simulink model "runQP"  (R2018a)
settings: Solver=VariableStepAuto  StartTime=0.0  StopTime=simTime  RelTol=1e-3
values from neighbouring files (symbols this model uses):
  Kd = 10    [com_notc.m]
  Kp = 200    [com_notc.m]
  q_initial_pos = robot.homeConfiguration    [com_notc.m]
undefined symbols (not defined in the file or in its folder): com_initial_pos
settings Model: Creator=yyakupoglu  LastModifiedBy=yyakupoglu

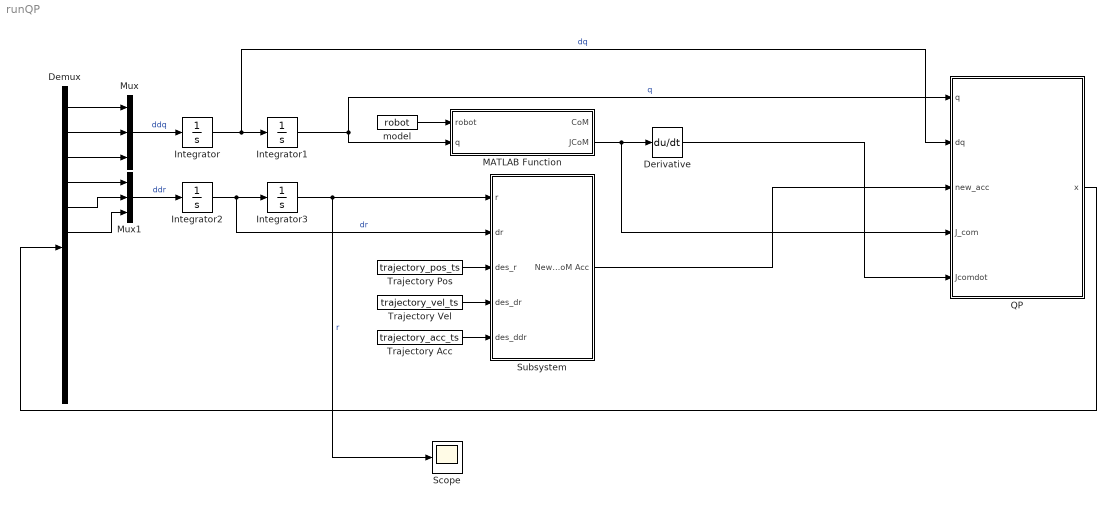
== system runQP ==
  Demux : Demux  Outputs=12
  Derivative : Derivative
  Integrator : Integrator  InitialCondition=[0;0;0]
  Integrator1 : Integrator  InitialCondition=q_initial_pos
  Integrator2 : Integrator  InitialCondition=[0;0;0]
  Integrator3 : Integrator  InitialCondition=com_initial_pos
  MATLAB Function : MATLAB Function  TreatAsAtomicUnit=on
  Mux : Mux  Inputs=3
  Mux1 : Mux  Inputs=3
  QP : MATLAB Function  TreatAsAtomicUnit=on
  Scope : Scope
  Subsystem : Subsystem
  Trajectory Acc : FromWorkspace  VariableName=trajectory_acc_ts  SampleTime=0
  Trajectory Pos : FromWorkspace  VariableName=trajectory_pos_ts  SampleTime=0
  Trajectory Vel : FromWorkspace  VariableName=trajectory_vel_ts  SampleTime=0
  model : FromWorkspace  VariableName=robot  SampleTime=0
  wires:
  Integrator/1 -> QP/2(dq), Integrator1/1  "dq"
  Demux/4 -> Mux1/1
  Demux/1 -> Mux/1
  Demux/2 -> Mux/2
  Demux/3 -> Mux/3
  Mux/1 -> Integrator/1  "ddq"
  Integrator1/1 -> MATLAB Function/2(q), QP/1(q)  "q"
  Demux/5 -> Mux1/2
  Mux1/1 -> Integrator2/1  "ddr"
  Integrator2/1 -> Subsystem/2(dr), Integrator3/1  "dr"
  Integrator3/1 -> Scope/1, Subsystem/1(r)  "r"
  MATLAB Function/2(JCoM) -> QP/4(J_com), Derivative/1
  Subsystem/1(New CoM Acc) -> QP/3(new_acc)
  Derivative/1 -> QP/5(Jcomdot)
  QP/1(x) -> Demux/1
  Demux/6 -> Mux1/3
  Trajectory Pos/1 -> Subsystem/3(des_r)
  Trajectory Vel/1 -> Subsystem/4(des_dr)
  Trajectory Acc/1 -> Subsystem/5(des_ddr)
  model/1 -> MATLAB Function/1(robot)

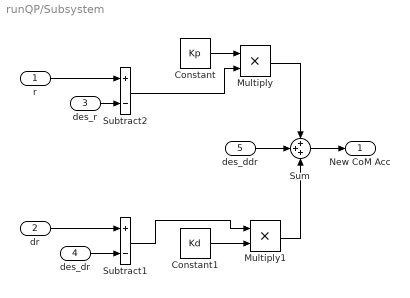
== system runQP/Subsystem ==
  r : Inport
  dr : Inport  Port=2
  des_r : Inport  Port=3
  des_dr : Inport  Port=4
  des_ddr : Inport  Port=5
  Constant : Constant  Value=Kp
  Constant1 : Constant  Value=Kd
  Multiply : Product
  Multiply1 : Product
  Subtract1 : Sum  Inputs=+-
  Subtract2 : Sum  Inputs=+-
  Sum : Sum  Inputs=+++
  New CoM Acc : Outport
  wires:
  r/1 -> Subtract2/1
  Sum/1 -> New CoM Acc/1
  Constant/1 -> Multiply/1
  Subtract2/1 -> Multiply/2
  Multiply/1 -> Sum/1
  Subtract1/1 -> Multiply1/1
  Constant1/1 -> Multiply1/2
  Multiply1/1 -> Sum/3
  des_r/1 -> Subtract2/2
  des_ddr/1 -> Sum/2
  dr/1 -> Subtract1/1
  des_dr/1 -> Subtract1/2

== matlab function runQP/MATLAB Function ==
  data: robot input; CoM output; JCoM output; q input
function [CoM, JCoM] = getCoMJacobian(robot,q)

[CoM, JCoM] = centerOfMass(robot,q)
end

== matlab function runQP/QP ==
  data: q input; x output; dq input; new_acc input; J_com input; Jcomdot input
function x = fcn(q, dq, new_acc, J_com, Jcomdot)
global robot m
J_dash=[-J_com eye(3)];
%Torque limit 
   tl=100; 
   nb=10^8;
   lb=[-nb,-nb,-nb,-nb,-nb,-nb,-tl,-tl,-tl,-nb,-nb,-nb];
   ub=[nb,nb,nb,nb,nb,nb,tl,tl,tl,nb,nb,nb];
   L=blkdiag(tl,tl,tl);
   
   
   
   %Dynamic Constraint Equations
   H=massMatrix(robot,q);
   M=blkdiag(H,eye(3)*(m));
   C=velocityProduct(robot,q,dq);
   G=gravityTorque(robot,q);
   hh=C+G;
   h = [hh;
         0;
         0];
     
S =[1 0 0 0 0 0;
       0 1 0 0 0 0;
       0 0 1 0 0 0];
   
   Jc=[0 0 0 1 0 0;
       0 0 0 0 1 0;
       0 0 0 0 0 1];
   A=[M -S' -Jc';
      J_dash zeros([3 6])];

   
   k=Jcomdot*dq;
   
   B=[-h;k];
   
   f=-[0;0;0;new_acc;0;0;0;0;0;0];
   
   
   W_diag = diag([0.0 0.0 0.0 1 1 1 0.0 0.0 0.0 0.0 0.0]);
   
   
   [x,fval,exitflag,output,lambda]=quadprog(W_diag,f,[],[],A,B,lb,ub,[],options);
end
